simulink model "synchro_v3"  (R2020b)
settings: Solver=FixedStepAuto  StartTime=0.0  StopTime=2  FixedStep=Ts  RelTol=1e-3
values from neighbouring files (symbols this model uses):
  m = 5/100    (= 0.05)    [synchro_parameters_v1.m]
  Sbase = 1    [synchro_parameters_v1.m]
  Ts = 1/Fs    (= 0.0001)    [synchro_parameters_v1.m]
  Vbase = 1    [synchro_parameters_v1.m]
  w_droop = 10*2*pi    (= 62.8318530718)    [synchro_parameters_v1.m]
  w_pll = 10*2*pi    (= 62.8318530718)    [synchro_parameters_v1.m]
  w_tau = 1e3*2*pi    (= 6283.18530718)    [synchro_parameters_v1.m]
  Wbase = 2*pi*50    (= 314.159265359)    [synchro_parameters_v1.m]
  Ybase = 1/Zbase    (= 1)    [synchro_parameters_v1.m]
  Zbase = Vbase/Ibase    (= 1)    [synchro_parameters_v1.m]
undefined symbols (not defined in the file or in its folder): DiscIntNeverNeededParam
libraries: SimplexPS x69, powerlib x64
(part 1 of 2)
settings Model: Creator=admin_user  LastModifiedBy=admin_user

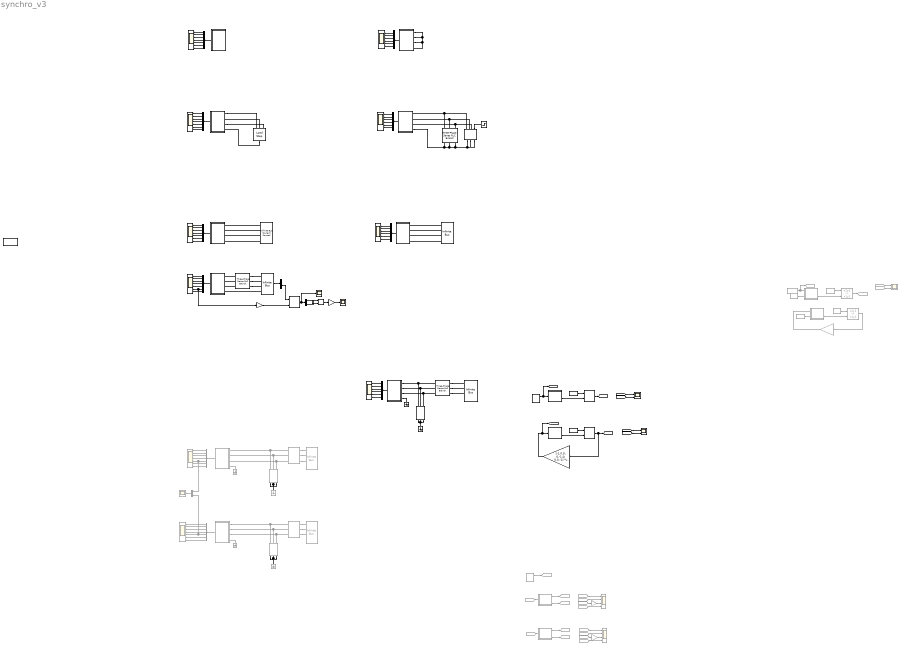
== system synchro_v3 ==
  note: Single-Inverter-Load System
  note: Droop inverter & voltage-source infinite bus
  note: PLL inverter & voltage-source infinite bus
  note: Droop inverter & current-source infinite bus
  note: Single-Inverter-Infinite-Bus System
  note: dq frame analysis
  note: PLL inverter + inifinite voltage bus (dq frame)
  note: PLL inverter + infinite voltage bus
  note: Droop analysis
  note: PLL analysis
  note: i-type
  note: Droop Inverter
  note: PLL inverter + R load
  note: PLL inverter & current-source infinite bus
  note: Droop inverter & R load
  note: PLL inverter & R load
  note: PLL inverter & R load
  note: Single-Inverter Extreme Operation
  note: Droop inverter & R load
  Atan : Trigonometry  Operator=atan2
  Bus Selector{,5,7,9} (4 alike) : BusSelector  OutputSignals=v_dq,i_dq,v_abc,i_abc,w,theta,pq
  Bus Selector1 : BusSelector  Commented=on  OutputSignals=v_dq,i_dq,v_abc,i_abc,w,theta,pq
  Bus Selector{3..4,8,10} (4 alike) : BusSelector  OutputSignals=v_dq,i_dq,v_abc,i_abc,w,theta
  Bus Selector2 : BusSelector  Commented=on  OutputSignals=v_dq,i_dq,v_abc,i_abc,w,theta,pq
  Bus Selector6 : BusSelector  OutputSignals=v_dq,v_abc
  Constant : Constant  Value=[1 0]
  Constant1 : Constant  Commented=on  Value=[1 0]
  Constant2 : Constant  Commented=on  Value=Wbase
  Constant3 : Constant  Commented=on  Value=[1 0]
  Constant4 : Constant  Value=[0.5 -0.1]
  Constant5 : Constant  Commented=on  Value=Wbase
  Constant6 : Constant  Commented=on  Value=[1;0]
  Demux : Demux  Outputs=2
  Droop Inverter : Subsystem
  Droop Inverter1 : Subsystem
  Droop Inverter2 : Subsystem
  Droop Inverter3 : Subsystem
  Frequency Droop (id) : Subsystem  Commented=on  AncestorBlock=SimplexPS/Frequency Droop (id)  mask{Ts=Ts, Sbase=Sbase, Vbase=Vbase, Wbase=Wbase, m=m, w_tau=w_droop, theta0=0, P0=0, W0=1}
      mask prompts: Ts "Ts (s), samping period"; Sbase "Sbase (VA), base power"; Vbase "Vbase (V), base voltage"; Wbase "Wbase (rad/s), base angular frequency"; m "m (pu), droop gain"; w_tau "w_tau (rad/s), low-pass filter bandwidth"; theta0 "theta0 (rad), initial angle"; P0 "P0 (pu), power setting point"; W0 "W0 (pu), frequency setting point"
  Frequency Droop (iq) : Subsystem  Commented=on  AncestorBlock=SimplexPS/Frequency Droop (iq)  mask{Ts=Ts, Sbase=Sbase, Vbase=Vbase, Wbase=Wbase, m=m, w_tau=w_droop, theta0=0, P0=0, W0=1}
      mask prompts: Ts "Ts (s), samping period"; Sbase "Sbase (VA), base power"; Vbase "Vbase (V), base voltage"; Wbase "Wbase (rad/s), base angular frequency"; m "m (pu), droop gain"; w_tau "w_tau (rad/s), low-pass filter bandwidth"; theta0 "theta0 (rad), initial angle"; P0 "P0 (pu), power setting point"; W0 "W0 (pu), frequency setting point"
  From{9..10,12,14} (4 alike) : From  Commented=on  GotoTag=i_abc3
  From11 : From  Commented=on  GotoTag=v_abc3
  From15 : From  Commented=on  GotoTag=v_abc4
  From16 : From  Commented=on  GotoTag=w4
  From17 : From  Commented=on  GotoTag=theta4
  From2 : From  Commented=on  GotoTag=vDQ_PLL
  From3 : From  Commented=on  GotoTag=iDQ_PLL
  From6 : From  Commented=on  GotoTag=w3
  From7 : From  Commented=on  GotoTag=theta3
  Gain : Gain  Commented=on  Gain=[0.5,0;0,0.5]  Multiplication=Matrix(K*u)
  Gain1 : Gain  Commented=on  Gain=1/Wbase
  Gain2 : Gain  Commented=on  Gain=1/Wbase
  Gain3 : Gain  Gain=[-1,0,0; 0,-1,0; 0,0,-1]  Multiplication=Matrix(K*u)
  Gain4 : Gain  Gain=2*pi
  Gain5 : Gain  Gain=1/(2*pi)
  Goto10 : Goto  Commented=on  GotoTag=theta4
  Goto2 : Goto  Commented=on  GotoTag=iDQ_PLL
  Goto3 : Goto  Commented=on  GotoTag=vDQ_PLL
  Goto5 : Goto  Commented=on  GotoTag=w3
  Goto6 : Goto  Commented=on  GotoTag=theta3
  Goto7 : Goto  Commented=on  GotoTag=i_abc3
  Goto9 : Goto  Commented=on  GotoTag=w4
  Ground{2..5} (4 alike) : powerlib/Elements/Ground  Commented=on  LConnTagsString=a
  Ground6 : powerlib/Elements/Ground  LConnTagsString=a
  Ground8 : powerlib/Elements/Ground  LConnTagsString=a
  Infinite Bus : SimplexPS/Infinite Bus  Commented=on  Ts=Ts  Sbase=Sbase  Vbase=Vbase  Wbase=Wbase  vd=1  vq=0  theta0=0  w=Wbase  R=1e-30
      settings: SourceProductName=Simplex Power Systems
  Infinite Bus (Current Source) : SimplexPS/Infinite Bus (Current Source)  Ts=Ts  Sbase=Sbase  Vbase=Vbase  Wbase=Wbase  id=1  iq=0  theta0=0  w=0.98
      settings: SourceProductName=Simplex Power Systems
  Infinite Bus1 : SimplexPS/Infinite Bus  Commented=on  Ts=Ts  Sbase=Sbase  Vbase=Vbase  Wbase=Wbase  vd=1  vq=0  theta0=0  w=Wbase  R=1e-30
      settings: SourceProductName=Simplex Power Systems
  Infinite Bus2 : SimplexPS/Infinite Bus  Ts=Ts  Sbase=Sbase  Vbase=Vbase  Wbase=Wbase  vd=1  vq=0  theta0=0  w=Wbase  R=1e-30
      settings: SourceProductName=Simplex Power Systems
  Infinite Bus3 : SimplexPS/Infinite Bus  Ts=Ts  Sbase=Sbase  Vbase=Vbase  Wbase=Wbase  vd=1  vq=0  theta0=0  w=Wbase  R=1e-30
      settings: SourceProductName=Simplex Power Systems
  Infinite Bus4 : SimplexPS/Infinite Bus  Ts=Ts  Sbase=Sbase  Vbase=Vbase  Wbase=Wbase  vd=1.01  vq=0  theta0=0  w=Wbase  R=1e-30
      settings: SourceProductName=Simplex Power Systems
  Load Step1 : SimplexPS/Load Step  t0=1  R=2*Zbase  Reverse=0
      settings: SourceProductName=Simplex Power Systems
  Mux : Mux  Commented=on  Inputs=2
  "PLL (vDQ -> vq)" : Subsystem  Commented=on  AncestorBlock=|  mask{Ts=Ts, Vbase=Vbase, Wbase=Wbase, w_PLL=w_pll, w_tau=w_tau, theta0=0}
      | SimplexPS/PLL
      | (vDQ -> vq)
      mask prompts: Ts "Ts (s), sampling period"; Vbase "Vbase (V), base voltage"; Wbase "Wbase (rad/s), base angular frequency"; w_PLL "w_pll (rad/s), PLL bandwidth"; w_tau "w_tau (rad/s), low-pass filter bandwidth"; theta0 "theta0 (rad), initial angle"
  "PLL (vDQ -> vq)1" : Subsystem  Commented=on  AncestorBlock=|  mask{Ts=Ts, Vbase=Vbase, Wbase=Wbase, w_PLL=w_pll, w_tau=w_tau, theta0=pi/2}
      | SimplexPS/PLL
      | (vDQ -> vq)
      mask prompts: Ts "Ts (s), sampling period"; Vbase "Vbase (V), base voltage"; Wbase "Wbase (rad/s), base angular frequency"; w_PLL "w_pll (rad/s), PLL bandwidth"; w_tau "w_tau (rad/s), low-pass filter bandwidth"; theta0 "theta0 (rad), initial angle"
  "PLL (vabc -> vq)" : Subsystem  AncestorBlock=|  mask{Ts=Ts, Vbase=Vbase, Wbase=Wbase, w_pll=w_pll, w_tau=w_tau, theta0=0}
      | SimplexPS/PLL
      | (vabc -> vq)
      mask prompts: Ts "Ts (s), sampling period"; Vbase "Vbase (V), base voltage"; Wbase "Wbase (rad/s), base angular frequency"; w_pll "w_pll (rad/s), PLL bandwidth"; w_tau "w_tau (rad/s), low-pass filter bandwidth"; theta0 "theta0 (rad), initial angle"
  "PLL (vabc -> vq)1" : Subsystem  AncestorBlock=|  mask{Ts=Ts, Vbase=Vbase, Wbase=Wbase, w_pll=w_pll, w_tau=w_tau, theta0=pi/2/2}
      | SimplexPS/PLL
      | (vabc -> vq)
      mask prompts: Ts "Ts (s), sampling period"; Vbase "Vbase (V), base voltage"; Wbase "Wbase (rad/s), base angular frequency"; w_pll "w_pll (rad/s), PLL bandwidth"; w_tau "w_tau (rad/s), low-pass filter bandwidth"; theta0 "theta0 (rad), initial angle"
  PLL Inverter : Subsystem
  PLL Inverter1 : Subsystem
  PLL Inverter2 : Subsystem
  PLL Inverter3 : Subsystem
  Scope{,11,14,16} (4 alike) : Scope  NumInputPorts=7
  Scope1 : Scope  NumInputPorts=2
  Scope{4,10,15,17} (4 alike) : Scope  NumInputPorts=6
  Scope12 : Scope
  Scope13 : Scope
  Scope2 : Scope  Commented=on  NumInputPorts=4
  Scope3 : Scope  Commented=on  NumInputPorts=7
  Scope5 : Scope  Commented=on  NumInputPorts=7
  Scope6 : Scope  Commented=on
  Scope7 : Scope  Commented=on  NumInputPorts=4
  Scope8 : Scope  Commented=on  NumInputPorts=2
  Scope9 : Scope  NumInputPorts=2
  Step : Step  SampleTime=0
  Three-Phase Parallel RLC Branch1 : powerlib/Elements/Three-Phase Parallel RLC Branch  Commented=on  LConnTagsString=A|B|C  RConnTagsString=A|B|C  BranchType=R  Resistance=1  Inductance=1e-3  Capacitance=1e-6  Measurements=None
      settings: SourceProductBaseCode=PS
  Three-Phase Parallel RLC Branch2 : powerlib/Elements/Three-Phase Parallel RLC Branch  Commented=on  LConnTagsString=A|B|C  RConnTagsString=A|B|C  BranchType=R  Resistance=1  Inductance=1e-3  Capacitance=1e-6  Measurements=None
      settings: SourceProductBaseCode=PS
  Three-Phase Series RLC Branch1 : powerlib/Elements/Three-Phase Series RLC Branch  LConnTagsString=A|B|C  RConnTagsString=A|B|C  BranchType=C  Resistance=1  Inductance=0.2/(2*pi*50)  Capacitance=Ybase*1e-3/Wbase  Measurements=None
  Three-Phase Series RLC Branch2 : powerlib/Elements/Three-Phase Series RLC Branch  Commented=on  LConnTagsString=A|B|C  RConnTagsString=A|B|C  BranchType=RL  Resistance=0.01  Inductance=0.2/(2*pi*50)  Capacitance=1e-6  Measurements=None
  Three-Phase Series RLC Branch3 : powerlib/Elements/Three-Phase Series RLC Branch  Commented=on  LConnTagsString=A|B|C  RConnTagsString=A|B|C  BranchType=RL  Resistance=0.01  Inductance=0.2/(2*pi*50)  Capacitance=1e-6  Measurements=None
  Three-Phase Series RLC Branch4 : powerlib/Elements/Three-Phase Series RLC Branch  LConnTagsString=A|B|C  RConnTagsString=A|B|C  BranchType=RL  Resistance=0.01*Zbase*0.4  Inductance=0.3*Zbase/Wbase*0.4  Capacitance=1/Wbase  Measurements=None
  Three-Phase Series RLC Branch5 : powerlib/Elements/Three-Phase Series RLC Branch  LConnTagsString=A|B|C  RConnTagsString=A|B|C  BranchType=RL  Resistance=0.3*Zbase/5  Inductance=0.3*Zbase/Wbase  Capacitance=1/Wbase  Measurements=None
  Three-Phase Series RLC Branch7 : powerlib/Elements/Three-Phase Series RLC Branch  LConnTagsString=A|B|C  RConnTagsString=A|B|C  BranchType=R  Resistance=2*Zbase  Inductance=0.3*Zbase/Wbase  Capacitance=1/Wbase  Measurements=None
  Three-Phase Breaker : powerlib/Elements/Three-Phase Breaker  InitialState=open  SwitchA=on  SwitchB=on  SwitchC=on  SwitchTimes="[1/60  5/60]"  External=on  BreakerResistance=1e-9  SnubberResistance=1e6  SnubberCapacitance=inf  Measurements=None
  Three-Phase Signal : SimplexPS/Three-Phase Signal  Commented=on  ud=1  uq=0  w=Wbase*1  theta0=0
      settings: SourceProductName=Simplex Power Systems
  Three-Phase Signal1 : SimplexPS/Three-Phase Signal  ud=1  uq=0  w=Wbase*0.95  theta0=pi/2/2
      settings: SourceProductName=Simplex Power Systems
  Voltage-Type Inverter (Droop)1 : Subsystem  Commented=on  mask{Sbase=Sbase, Vbase=Vbase, Wbase=Wbase, Ts=Ts, v_d0=1, v_q0=0, w0=1, m=m, n=0, P0=0, Q0=0, w_droop=w_droop}
      mask prompts: Sbase "Sbase (VA)"; Vbase "Vbase (V)"; Wbase "Wbase (rad/s)"; Ts "Ts (s)"; v_d0 "v_d0 (pu), d-axis voltage setting point"; v_q0 "v_q0 (pu), q-axis voltage setting point"; w0 "w0 (pu), frequency setting point"; m "m (pu), frequency droop gain"; n "n (pu), voltage droop gain"; P0 "P0 (pu), active power setting point"; Q0 "Q0 (pu), reactive power setting point"; w_droop "w_droop (rad/s), droop bandwidth"
  Voltage-Type Inverter (Droop)2 : Subsystem  Commented=on  mask{Sbase=Sbase, Vbase=Vbase, Wbase=Wbase, Ts=Ts, v_d0=1, v_q0=0, w0=1, m=m, n=0, P0=0, Q0=0, w_droop=w_droop}
      mask prompts: Sbase "Sbase (VA)"; Vbase "Vbase (V)"; Wbase "Wbase (rad/s)"; Ts "Ts (s)"; v_d0 "v_d0 (pu), d-axis voltage setting point"; v_q0 "v_q0 (pu), q-axis voltage setting point"; w0 "w0 (pu), frequency setting point"; m "m (pu), frequency droop gain"; n "n (pu), voltage droop gain"; P0 "P0 (pu), active power setting point"; Q0 "Q0 (pu), reactive power setting point"; w_droop "w_droop (rad/s), droop bandwidth"
  "abc -> dq (Power-Invariant)" : SimplexPS/abc -> dq (Power-Invariant)  SystemSampleTime=-1  VariantActivationTime=update diagram  Latency=0  AutoFrameSizeCalculation=off
      settings: SourceProductName=Simplex Power Systems
  "dq -> abc (Power-Invariant)" : SimplexPS/dq -> abc (Power-Invariant)  SystemSampleTime=-1  VariantActivationTime=update diagram  Latency=0  AutoFrameSizeCalculation=off
      settings: SourceProductName=Simplex Power Systems
  "dq -> abc (Power-Invariant)1" : SimplexPS/dq -> abc (Power-Invariant)  SystemSampleTime=-1  VariantActivationTime=update diagram  Latency=0  AutoFrameSizeCalculation=off
      settings: SourceProductName=Simplex Power Systems
  powergui : powerlib/powergui  Priority=1  SimulationMode=Discrete  SampleTime=Ts  frequency=60  Iterations=50  frequencyindice=0  Pbase=100e6  ErrMax=1e-4  UnitsV=kV  UnitsW=MW  buscounter=0  FunctionMessages=off  echomessages=off  EnableUseOfTLC=off  CurrentSourceSwitches=off  DisableSnubberDevices=off  DisableRonSwitches=off  DisableVfSwitches=off  DisplayEquations=off  AutomaticDiscreteSolvers=off  SolverType=Tustin/Backward Euler (TBE)  Interpol=off  ExternalGateDelay=off  methode=off  Ts=100  x0status=blocks  SPID=on  SwTol=0  HookPort=off  NonlinearTolerance=1e-4  nMaxIteration=100  ContinueOnMaxIteration=off  RestoreLinks=warning  ResistiveCurrentMeasurement=off  Frange=[0:2:500]  Ylog=off  Xlog=on  ShowGrid=off  save=off  variable=ZData  structure=0  ZoomFFT=off  StartTime=0.0  cycles=1  DisplayStyle=1  fundamental=60  FreqAxis=off  MaxFrequency=1000  frequencyindicesteady=1  RmsSteady=1  display=off
  "x2y2 -> x1y1" : SimplexPS/x2y2 -> x1y1  Commented=on  SystemSampleTime=-1  VariantActivationTime=update diagram  Latency=0  AutoFrameSizeCalculation=off
      settings: SourceProductName=Simplex Power Systems
  "x2y2 -> x1y2" : SimplexPS/x2y2 -> x1y1  Commented=on  SystemSampleTime=-1  VariantActivationTime=update diagram  Latency=0  AutoFrameSizeCalculation=off
      settings: SourceProductName=Simplex Power Systems
  wires:
  Droop Inverter/1(m) -> Bus Selector/1
  Bus Selector/1 -> Scope/1  "<v_dq>"
  Bus Selector/2 -> Scope/2  "<i_dq>"
  Bus Selector/3 -> Scope/3  "<v_abc>"
  Bus Selector/4 -> Scope/4  "<i_abc>"
  Bus Selector/5 -> Scope/5  "<w>"
  Bus Selector/6 -> Scope/6  "<theta>"
  Bus Selector/7 -> Scope/7  "<pq>"
  Bus Selector4/3 -> Scope4/3  "<v_abc>"
  Bus Selector4/4 -> Scope4/4  "<i_abc>"
  Bus Selector4/6 -> Scope4/6  "<theta>"
  Bus Selector4/1 -> Scope4/1  "<v_dq>"
  PLL Inverter/1(m) -> Bus Selector4/1
  Bus Selector4/5 -> Scope4/5  "<w>"
  Bus Selector4/2 -> Scope4/2  "<i_dq>"
  Frequency Droop (id)/1(w) -> Goto5/1
  Frequency Droop (id)/3(theta) -> Goto6/1
  From7/1 -> Scope2/4
  Three-Phase Signal/1 -> Goto7/1
  From9/1 -> Frequency Droop (id)/1(iabc)
  From10/1 -> Scope2/1
  From11/1 -> Scope2/2
  From6/1 -> Gain1/1
  Gain1/1 -> Scope2/3
  Bus Selector1/5 -> Mux/1, Scope3/5  "<w>"
  Bus Selector1/3 -> Scope3/3  "<v_abc>"
  Bus Selector1/6 -> Scope3/6  "<theta>"
  Bus Selector1/7 -> Scope3/7  "<pq>"
  Bus Selector1/2 -> Scope3/2  "<i_dq>"
  Bus Selector1/4 -> Scope3/4  "<i_abc>"
  Bus Selector1/1 -> Scope3/1  "<v_dq>"
  Voltage-Type Inverter (Droop)1/1(m) -> Bus Selector1/1
  Bus Selector2/2 -> Scope5/2  "<i_dq>"
  Bus Selector2/4 -> Scope5/4  "<i_abc>"
  Bus Selector2/1 -> Scope5/1  "<v_dq>"
  Voltage-Type Inverter (Droop)2/1(m) -> Bus Selector2/1
  Bus Selector2/6 -> Scope5/6  "<theta>"
  Bus Selector2/3 -> Scope5/3  "<v_abc>"
  Bus Selector2/7 -> Scope5/7  "<pq>"
  Bus Selector2/5 -> Mux/2, Scope5/5  "<w>"
  Mux/1 -> Scope6/1
  From12/1 -> Frequency Droop (iq)/1(iabc)
  Frequency Droop (iq)/1(w) -> Goto9/1
  Frequency Droop (iq)/3(theta) -> Goto10/1
  From17/1 -> Scope7/4
  From16/1 -> Gain2/1
  From15/1 -> Scope7/2
  From14/1 -> Scope7/1
  Gain2/1 -> Scope7/3
  Three-Phase Signal1/1 -> "PLL (vabc -> vq)"/1(vabc), [vabc_PLL1]
  Constant/1 -> "dq -> abc (Power-Invariant)"/1
  "PLL (vabc -> vq)"/2(theta) -> "dq -> abc (Power-Invariant)"/2
  "dq -> abc (Power-Invariant)"/1 -> [iabc_PLL1]
  [iabc_PLL1] -> Scope1/2
  [vabc_PLL1] -> Scope1/1
  Constant2/1 -> "PLL (vDQ -> vq)"/2(wDQ)
  Constant3/1 -> "x2y2 -> x1y1"/1
  "PLL (vDQ -> vq)"/2(theta) -> "x2y2 -> x1y1"/2
  "x2y2 -> x1y1"/1 -> Goto2/1
  Constant1/1 -> "PLL (vDQ -> vq)"/1(vDQ), Goto3/1
  From2/1 -> Scope8/1
  From3/1 -> Scope8/2
  Constant6/1 -> "x2y2 -> x1y2"/1
  "PLL (vDQ -> vq)1"/2(theta) -> "x2y2 -> x1y2"/2
  "x2y2 -> x1y2"/1 -> Gain/1
  Constant5/1 -> "PLL (vDQ -> vq)1"/2(wDQ)
  Gain/1 -> "PLL (vDQ -> vq)1"/1(vDQ)
  "PLL (vabc -> vq)1"/2(theta) -> "dq -> abc (Power-Invariant)1"/2
  [vabc_PLL2] -> Scope9/1
  Constant4/1 -> "dq -> abc (Power-Invariant)1"/1
  Gain3/1 -> [vabc_PLL2], "PLL (vabc -> vq)1"/1(vabc)
  [iabc_PLL2] -> Scope9/2
  "dq -> abc (Power-Invariant)1"/1 -> [iabc_PLL2], Gain3/1
  Bus Selector3/3 -> Scope10/3  "<v_abc>"
  Bus Selector3/1 -> Scope10/1  "<v_dq>"
  Bus Selector3/6 -> Scope10/6  "<theta>"
  Bus Selector3/5 -> Scope10/5  "<w>"
  Bus Selector3/4 -> Scope10/4  "<i_abc>"
  PLL Inverter1/1(m) -> Bus Selector3/1
  Bus Selector3/2 -> Scope10/2  "<i_dq>"
  Bus Selector5/1 -> Scope11/1  "<v_dq>"
  Bus Selector5/6 -> Gain4/1, Scope11/6  "<theta>"
  Bus Selector5/2 -> Scope11/2  "<i_dq>"
  Bus Selector5/4 -> Scope11/4  "<i_abc>"
  Droop Inverter1/1(m) -> Bus Selector5/1
  Bus Selector5/7 -> Scope11/7  "<pq>"
  Bus Selector5/5 -> Scope11/5  "<w>"
  Bus Selector5/3 -> Scope11/3  "<v_abc>"
  Infinite Bus4/1 -> Bus Selector6/1
  Bus Selector6/2 -> "abc -> dq (Power-Invariant)"/1  "<v_abc>"
  Demux/1 -> Atan/2
  Demux/2 -> Atan/1
  "abc -> dq (Power-Invariant)"/1 -> Scope13/1, Demux/1
  Gain4/1 -> "abc -> dq (Power-Invariant)"/2
  Atan/1 -> Gain5/1
  Gain5/1 -> Scope12/1
  Bus Selector7/3 -> Scope14/3  "<v_abc>"
  Bus Selector7/6 -> Scope14/6  "<theta>"
  Bus Selector7/2 -> Scope14/2  "<i_dq>"
  Bus Selector7/1 -> Scope14/1  "<v_dq>"
  Droop Inverter2/1(m) -> Bus Selector7/1
  Bus Selector7/7 -> Scope14/7  "<pq>"
  Bus Selector7/5 -> Scope14/5  "<w>"
  Bus Selector7/4 -> Scope14/4  "<i_abc>"
  PLL Inverter2/1(m) -> Bus Selector8/1
  Bus Selector8/2 -> Scope15/2  "<i_dq>"
  Bus Selector8/1 -> Scope15/1  "<v_dq>"
  Bus Selector8/4 -> Scope15/4  "<i_abc>"
  Bus Selector8/3 -> Scope15/3  "<v_abc>"
  Bus Selector8/6 -> Scope15/6  "<theta>"
  Bus Selector8/5 -> Scope15/5  "<w>"
  Bus Selector10/4 -> Scope17/4  "<i_abc>"
  Bus Selector10/5 -> Scope17/5  "<w>"
  PLL Inverter3/1(m) -> Bus Selector10/1
  Bus Selector9/5 -> Scope16/5  "<w>"
  Bus Selector9/1 -> Scope16/1  "<v_dq>"
  Bus Selector10/6 -> Scope17/6  "<theta>"
  Bus Selector9/7 -> Scope16/7  "<pq>"
  Bus Selector9/2 -> Scope16/2  "<i_dq>"
  Bus Selector10/1 -> Scope17/1  "<v_dq>"
  Bus Selector9/4 -> Scope16/4  "<i_abc>"
  Droop Inverter3/1(m) -> Bus Selector9/1
  Bus Selector9/6 -> Scope16/6  "<theta>"
  Bus Selector9/3 -> Scope16/3  "<v_abc>"
  Bus Selector10/2 -> Scope17/2  "<i_dq>"
  Bus Selector10/3 -> Scope17/3  "<v_abc>"
  Step/1 -> Three-Phase Breaker/1
  connections:
  Infinite Bus (Current Source)/LConn1 -- Droop Inverter/LConn1
  Infinite Bus (Current Source)/LConn2 -- Droop Inverter/LConn2
  Infinite Bus (Current Source)/LConn3 -- Droop Inverter/LConn3
  PLL Inverter/LConn4 -- Ground8/LConn1
  Three-Phase Parallel RLC Branch1/RConn2 -- Ground2/LConn1 -- Three-Phase Parallel RLC Branch1/RConn3 -- Three-Phase Parallel RLC Branch1/RConn1
  Three-Phase Parallel RLC Branch1/LConn3 -- Voltage-Type Inverter (Droop)1/LConn3 -- Three-Phase Series RLC Branch3/LConn3
  Ground3/LConn1 -- Voltage-Type Inverter (Droop)1/LConn4
  Three-Phase Parallel RLC Branch1/LConn2 -- Voltage-Type Inverter (Droop)1/LConn2 -- Three-Phase Series RLC Branch3/LConn2
  Three-Phase Parallel RLC Branch1/LConn1 -- Voltage-Type Inverter (Droop)1/LConn1 -- Three-Phase Series RLC Branch3/LConn1
  Three-Phase Parallel RLC Branch2/RConn2 -- Ground4/LConn1 -- Three-Phase Parallel RLC Branch2/RConn3 -- Three-Phase Parallel RLC Branch2/RConn1
  Voltage-Type Inverter (Droop)2/LConn3 -- Three-Phase Series RLC Branch2/LConn3 -- Three-Phase Parallel RLC Branch2/LConn3
  Ground5/LConn1 -- Voltage-Type Inverter (Droop)2/LConn4
  Voltage-Type Inverter (Droop)2/LConn1 -- Three-Phase Parallel RLC Branch2/LConn1 -- Three-Phase Series RLC Branch2/LConn1
  Voltage-Type Inverter (Droop)2/LConn2 -- Three-Phase Series RLC Branch2/LConn2 -- Three-Phase Parallel RLC Branch2/LConn2
  Three-Phase Series RLC Branch2/RConn1 -- Infinite Bus/LConn1
  Three-Phase Series RLC Branch2/RConn2 -- Infinite Bus/LConn2
  Three-Phase Series RLC Branch2/RConn3 -- Infinite Bus/LConn3
  Three-Phase Series RLC Branch3/RConn1 -- Infinite Bus1/LConn1
  Three-Phase Series RLC Branch3/RConn3 -- Infinite Bus1/LConn3
  Three-Phase Series RLC Branch3/RConn2 -- Infinite Bus1/LConn2
  Ground6/LConn1 -- Three-Phase Series RLC Branch1/RConn3 -- Three-Phase Series RLC Branch1/RConn2 -- Three-Phase Series RLC Branch1/RConn1
  PLL Inverter/LConn1 -- Three-Phase Series RLC Branch1/LConn1 -- Three-Phase Series RLC Branch4/RConn1
  PLL Inverter/LConn2 -- Three-Phase Series RLC Branch1/LConn2 -- Three-Phase Series RLC Branch4/RConn2
  PLL Inverter/LConn3 -- Three-Phase Series RLC Branch4/RConn3 -- Three-Phase Series RLC Branch1/LConn3
  Three-Phase Series RLC Branch4/LConn1 -- Infinite Bus2/LConn1
  Three-Phase Series RLC Branch4/LConn2 -- Infinite Bus2/LConn2
  Three-Phase Series RLC Branch4/LConn3 -- Infinite Bus2/LConn3
  Infinite Bus3/LConn1 -- PLL Inverter1/LConn1
  Infinite Bus3/LConn2 -- PLL Inverter1/LConn2
  Infinite Bus3/LConn3 -- PLL Inverter1/LConn3
  Infinite Bus3/LConn4 -- PLL Inverter1/LConn4
  Infinite Bus (Current Source)/LConn4 -- Droop Inverter/LConn4
  Infinite Bus4/LConn4 -- Droop Inverter1/LConn4
  Three-Phase Series RLC Branch5/RConn1 -- Droop Inverter1/LConn1
  Three-Phase Series RLC Branch5/RConn2 -- Droop Inverter1/LConn2
  Three-Phase Series RLC Branch5/RConn3 -- Droop Inverter1/LConn3
  Three-Phase Series RLC Branch5/LConn1 -- Infinite Bus4/LConn1
  Three-Phase Series RLC Branch5/LConn2 -- Infinite Bus4/LConn2
  Three-Phase Series RLC Branch5/LConn3 -- Infinite Bus4/LConn3
  Droop Inverter2/LConn1 -- Load Step1/LConn1
  Load Step1/LConn2 -- Droop Inverter2/LConn2
  Droop Inverter2/LConn3 -- Load Step1/LConn3
  Load Step1/RConn1 -- Droop Inverter2/LConn4
  Three-Phase Series RLC Branch7/RConn1 -- Three-Phase Breaker/LConn3 -- PLL Inverter2/LConn1
  Three-Phase Series RLC Branch7/RConn2 -- Three-Phase Breaker/LConn2 -- PLL Inverter2/LConn2
  Three-Phase Series RLC Branch7/RConn3 -- Three-Phase Breaker/LConn1 -- PLL Inverter2/LConn3
  PLL Inverter2/LConn4 -- Three-Phase Breaker/RConn1 -- Three-Phase Breaker/RConn2 -- Three-Phase Breaker/RConn3 -- Three-Phase Series RLC Branch7/LConn3 -- Three-Phase Series RLC Branch7/LConn2 -- Three-Phase Series RLC Branch7/LConn1
  PLL Inverter3/LConn1 -- PLL Inverter3/LConn2 -- PLL Inverter3/LConn3 -- PLL Inverter3/LConn4

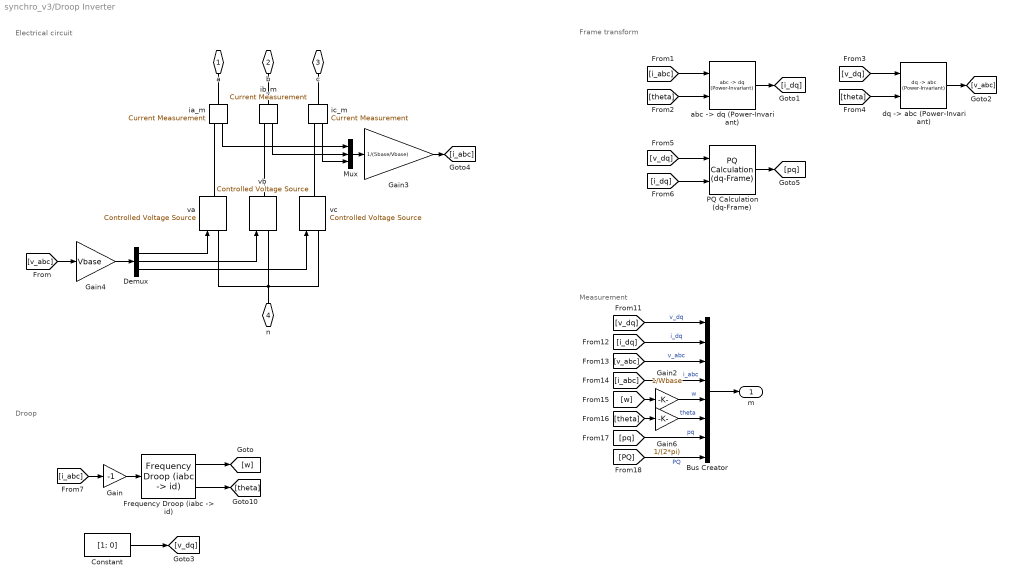
== system synchro_v3/Droop Inverter ==
  note: Measurement
  note: Droop
  note: Frame transform
  note: Electrical circuit
  Bus Creator : BusCreator  Inputs=8
  Constant : Constant  Value=[1; 0]
  Demux : Demux  Outputs=3
  "Frequency Droop (iabc -> id)" : SimplexPS/Frequency Droop (iabc -> id)  Ts=Ts  Sbase=Sbase  Vbase=Vbase  Wbase=Wbase  m=m  w_tau=w_droop  theta0=0  i0=0  w0=1
      settings: SourceProductName=Simplex Power Systems
  Gain : Gain  Gain=-1
  Gain2 : Gain  Gain=1/Wbase
  Gain3 : Gain  Gain=1/(Sbase/Vbase)
  Gain4 : Gain  Gain=Vbase
  Gain6 : Gain  Gain=1/(2*pi)
  Mux : Mux  Inputs=3
  PQ Calculation (dq-Frame) : SimplexPS/PQ Calculation (dq-Frame)  SystemSampleTime=-1  VariantActivationTime=update diagram  Latency=0  AutoFrameSizeCalculation=off
      settings: SourceProductName=Simplex Power Systems
  "abc -> dq (Power-Invariant)" : SimplexPS/abc -> dq (Power-Invariant)  SystemSampleTime=-1  VariantActivationTime=update diagram  Latency=0  AutoFrameSizeCalculation=off
      settings: SourceProductName=Simplex Power Systems
  "dq -> abc (Power-Invariant)" : SimplexPS/dq -> abc (Power-Invariant)  SystemSampleTime=-1  VariantActivationTime=update diagram  Latency=0  AutoFrameSizeCalculation=off
      settings: SourceProductName=Simplex Power Systems
  ia_m : powerlib/Measurements/Current Measurement  PhasorSimulation=off  OutputType=Complex  PSBequivalent=0
  ib_m : powerlib/Measurements/Current Measurement  PhasorSimulation=off  OutputType=Complex  PSBequivalent=0
  ic_m : powerlib/Measurements/Current Measurement  PhasorSimulation=off  OutputType=Complex  PSBequivalent=0
  va : powerlib/Electrical Sources/Controlled Voltage Source  Initialize=on  Source_Type=AC  Amplitude=0  Phase=0  Frequency=0  Measurements=None
  vb : powerlib/Electrical Sources/Controlled Voltage Source  Initialize=on  Source_Type=AC  Amplitude=0  Phase=0  Frequency=0  Measurements=None
  vc : powerlib/Electrical Sources/Controlled Voltage Source  Initialize=on  Source_Type=AC  Amplitude=0  Phase=0  Frequency=0  Measurements=None
  a : PMIOPort  Side=Left
  b : PMIOPort  Port=2  Side=Left
  c : PMIOPort  Port=3  Side=Left
  n : PMIOPort  Port=4  Side=Left
  m : Outport
  wires:
  ic_m/1 -> Mux/3
  ia_m/1 -> Mux/1
  ib_m/1 -> Mux/2
  Demux/1 -> va/1
  Demux/2 -> vb/1
  Demux/3 -> vc/1
  [i_abc] -> "abc -> dq (Power-Invariant)"/1
  [theta] -> "abc -> dq (Power-Invariant)"/2
  "abc -> dq (Power-Invariant)"/1 -> [i_dq]
  [v_dq] -> "dq -> abc (Power-Invariant)"/1
  [theta] -> "dq -> abc (Power-Invariant)"/2
  "dq -> abc (Power-Invariant)"/1 -> [v_abc]
  [v_dq] -> Bus Creator/1  "v_dq"
  [v_abc] -> Bus Creator/3  "v_abc"
  [i_abc] -> Bus Creator/4  "i_abc"
  [pq] -> Bus Creator/7  "pq"
  [PQ] -> Bus Creator/8  "PQ"
  Bus Creator/1 -> m/1
  [w] -> Gain2/1
  Gain2/1 -> Bus Creator/5  "w"
  Mux/1 -> Gain3/1
  Gain3/1 -> [i_abc]
  [v_abc] -> Gain4/1
  Gain4/1 -> Demux/1
  [theta] -> Gain6/1
  Gain6/1 -> Bus Creator/6  "theta"
  "Frequency Droop (iabc -> id)"/2 -> [theta]
  [i_abc] -> Gain/1
  "Frequency Droop (iabc -> id)"/1 -> [w]
  Constant/1 -> [v_dq]
  [i_dq] -> Bus Creator/2  "i_dq"
  [v_dq] -> PQ Calculation (dq-Frame)/1
  [i_dq] -> PQ Calculation (dq-Frame)/2
  PQ Calculation (dq-Frame)/1 -> [pq]
  Gain/1 -> "Frequency Droop (iabc -> id)"/1
  connections:
  ia_m/RConn1 -- va/RConn1
  ia_m/LConn1 -- a/RConn1
  ib_m/RConn1 -- vb/RConn1
  ic_m/RConn1 -- vc/RConn1
  va/LConn1 -- vb/LConn1 -- vc/LConn1 -- n/RConn1
  ib_m/LConn1 -- b/RConn1
  ic_m/LConn1 -- c/RConn1

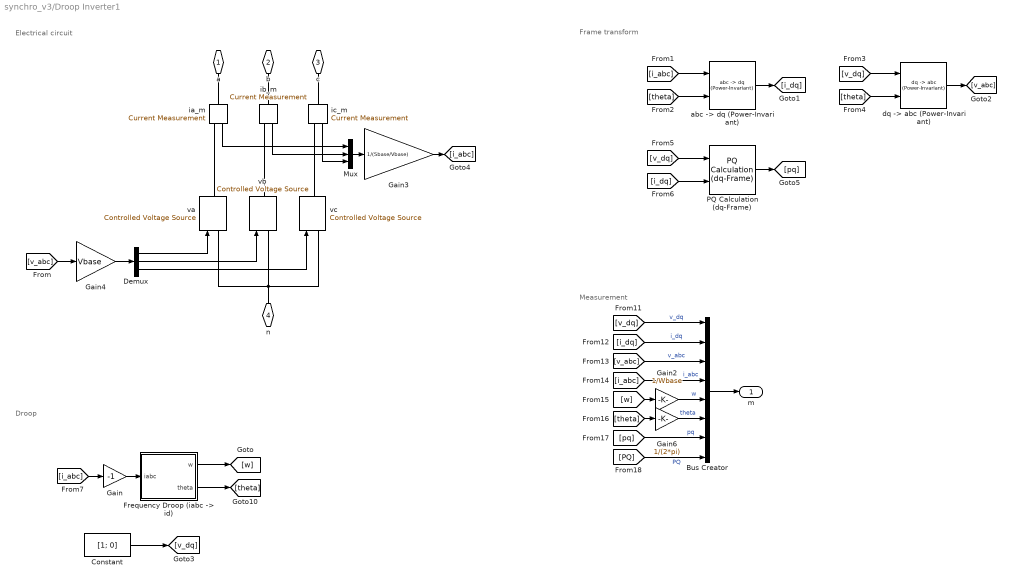
== system synchro_v3/Droop Inverter1 ==
  note: Measurement
  note: Droop
  note: Frame transform
  note: Electrical circuit
  Bus Creator : BusCreator  Inputs=8
  Constant : Constant  Value=[1; 0]
  Demux : Demux  Outputs=3
  "Frequency Droop (iabc -> id)" : Subsystem  AncestorBlock=|  mask{Ts=Ts, Sbase=Sbase, Vbase=Vbase, Wbase=Wbase, m=m, w_tau=w_droop, theta0=0, i0=0, w0=1}
      | SimplexPS/Frequency Droop
      | (iabc -> id)
      mask prompts: Ts "Ts (s), samping period"; Sbase "Sbase (VA), base power"; Vbase "Vbase (V), base voltage"; Wbase "Wbase (rad/s), base angular frequency"; m "m (pu), droop gain"; w_tau "w_tau (rad/s), low-pass filter bandwidth"; theta0 "theta0 (rad), initial angle"; i0 "i0 (pu), current setting point"; w0 "w0 (pu), frequency setting point"
  Gain : Gain  Gain=-1
  Gain2 : Gain  Gain=1/Wbase
  Gain3 : Gain  Gain=1/(Sbase/Vbase)
  Gain4 : Gain  Gain=Vbase
  Gain6 : Gain  Gain=1/(2*pi)
  Mux : Mux  Inputs=3
  PQ Calculation (dq-Frame) : SimplexPS/PQ Calculation (dq-Frame)  SystemSampleTime=-1  VariantActivationTime=update diagram  Latency=0  AutoFrameSizeCalculation=off
      settings: SourceProductName=Simplex Power Systems
  "abc -> dq (Power-Invariant)" : SimplexPS/abc -> dq (Power-Invariant)  SystemSampleTime=-1  VariantActivationTime=update diagram  Latency=0  AutoFrameSizeCalculation=off
      settings: SourceProductName=Simplex Power Systems
  "dq -> abc (Power-Invariant)" : SimplexPS/dq -> abc (Power-Invariant)  SystemSampleTime=-1  VariantActivationTime=update diagram  Latency=0  AutoFrameSizeCalculation=off
      settings: SourceProductName=Simplex Power Systems
  ia_m : powerlib/Measurements/Current Measurement  PhasorSimulation=off  OutputType=Complex  PSBequivalent=0
  ib_m : powerlib/Measurements/Current Measurement  PhasorSimulation=off  OutputType=Complex  PSBequivalent=0
  ic_m : powerlib/Measurements/Current Measurement  PhasorSimulation=off  OutputType=Complex  PSBequivalent=0
  va : powerlib/Electrical Sources/Controlled Voltage Source  Initialize=on  Source_Type=AC  Amplitude=0  Phase=0  Frequency=0  Measurements=None
  vb : powerlib/Electrical Sources/Controlled Voltage Source  Initialize=on  Source_Type=AC  Amplitude=0  Phase=0  Frequency=0  Measurements=None
  vc : powerlib/Electrical Sources/Controlled Voltage Source  Initialize=on  Source_Type=AC  Amplitude=0  Phase=0  Frequency=0  Measurements=None
  a : PMIOPort  Side=Left
  b : PMIOPort  Port=2  Side=Left
  c : PMIOPort  Port=3  Side=Left
  n : PMIOPort  Port=4  Side=Left
  m : Outport
  wires:
  ic_m/1 -> Mux/3
  ia_m/1 -> Mux/1
  ib_m/1 -> Mux/2
  Demux/1 -> va/1
  Demux/2 -> vb/1
  Demux/3 -> vc/1
  [i_abc] -> "abc -> dq (Power-Invariant)"/1
  [theta] -> "abc -> dq (Power-Invariant)"/2
  "abc -> dq (Power-Invariant)"/1 -> [i_dq]
  [v_dq] -> "dq -> abc (Power-Invariant)"/1
  [theta] -> "dq -> abc (Power-Invariant)"/2
  "dq -> abc (Power-Invariant)"/1 -> [v_abc]
  [v_dq] -> Bus Creator/1  "v_dq"
  [v_abc] -> Bus Creator/3  "v_abc"
  [i_abc] -> Bus Creator/4  "i_abc"
  [pq] -> Bus Creator/7  "pq"
  [PQ] -> Bus Creator/8  "PQ"
  Bus Creator/1 -> m/1
  [w] -> Gain2/1
  Gain2/1 -> Bus Creator/5  "w"
  Mux/1 -> Gain3/1
  Gain3/1 -> [i_abc]
  [v_abc] -> Gain4/1
  Gain4/1 -> Demux/1
  [theta] -> Gain6/1
  Gain6/1 -> Bus Creator/6  "theta"
  "Frequency Droop (iabc -> id)"/2(theta) -> [theta]
  [i_abc] -> Gain/1
  "Frequency Droop (iabc -> id)"/1(w) -> [w]
  Constant/1 -> [v_dq]
  [i_dq] -> Bus Creator/2  "i_dq"
  [v_dq] -> PQ Calculation (dq-Frame)/1
  [i_dq] -> PQ Calculation (dq-Frame)/2
  PQ Calculation (dq-Frame)/1 -> [pq]
  Gain/1 -> "Frequency Droop (iabc -> id)"/1(iabc)
  connections:
  ia_m/RConn1 -- va/RConn1
  ia_m/LConn1 -- a/RConn1
  ib_m/RConn1 -- vb/RConn1
  ic_m/RConn1 -- vc/RConn1
  va/LConn1 -- vb/LConn1 -- vc/LConn1 -- n/RConn1
  ib_m/LConn1 -- b/RConn1
  ic_m/LConn1 -- c/RConn1

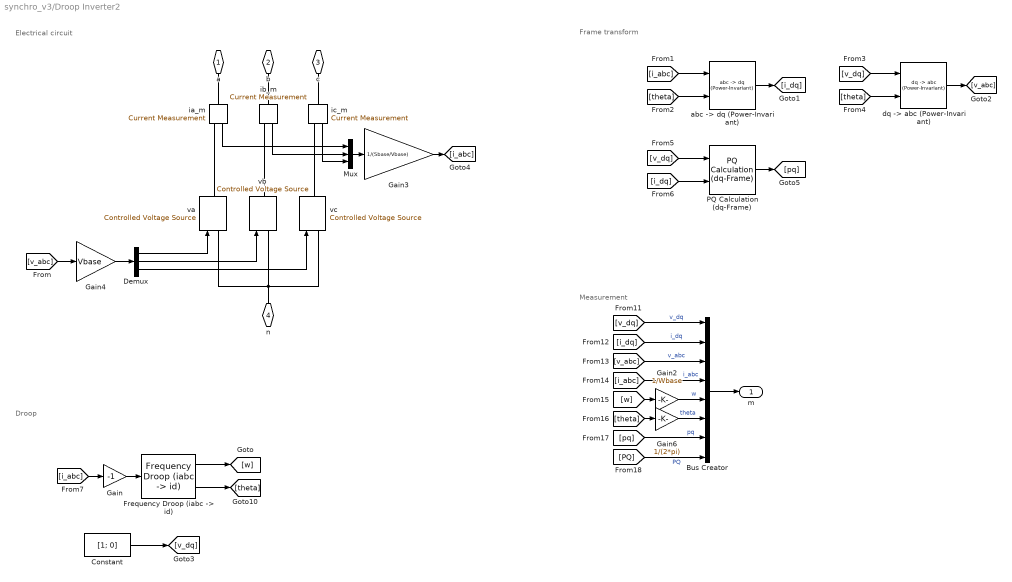
== system synchro_v3/Droop Inverter2 ==
  note: Measurement
  note: Droop
  note: Frame transform
  note: Electrical circuit
  Bus Creator : BusCreator  Inputs=8
  Constant : Constant  Value=[1; 0]
  Demux : Demux  Outputs=3
  "Frequency Droop (iabc -> id)" : SimplexPS/Frequency Droop (iabc -> id)  Ts=Ts  Sbase=Sbase  Vbase=Vbase  Wbase=Wbase  m=m  w_tau=w_droop  theta0=0  i0=0  w0=1
      settings: SourceProductName=Simplex Power Systems
  Gain : Gain  Gain=-1
  Gain2 : Gain  Gain=1/Wbase
  Gain3 : Gain  Gain=1/(Sbase/Vbase)
  Gain4 : Gain  Gain=Vbase
  Gain6 : Gain  Gain=1/(2*pi)
  Mux : Mux  Inputs=3
  PQ Calculation (dq-Frame) : SimplexPS/PQ Calculation (dq-Frame)  SystemSampleTime=-1  VariantActivationTime=update diagram  Latency=0  AutoFrameSizeCalculation=off
      settings: SourceProductName=Simplex Power Systems
  "abc -> dq (Power-Invariant)" : SimplexPS/abc -> dq (Power-Invariant)  SystemSampleTime=-1  VariantActivationTime=update diagram  Latency=0  AutoFrameSizeCalculation=off
      settings: SourceProductName=Simplex Power Systems
  "dq -> abc (Power-Invariant)" : SimplexPS/dq -> abc (Power-Invariant)  SystemSampleTime=-1  VariantActivationTime=update diagram  Latency=0  AutoFrameSizeCalculation=off
      settings: SourceProductName=Simplex Power Systems
  ia_m : powerlib/Measurements/Current Measurement  PhasorSimulation=off  OutputType=Complex  PSBequivalent=0
  ib_m : powerlib/Measurements/Current Measurement  PhasorSimulation=off  OutputType=Complex  PSBequivalent=0
  ic_m : powerlib/Measurements/Current Measurement  PhasorSimulation=off  OutputType=Complex  PSBequivalent=0
  va : powerlib/Electrical Sources/Controlled Voltage Source  Initialize=on  Source_Type=AC  Amplitude=0  Phase=0  Frequency=0  Measurements=None
  vb : powerlib/Electrical Sources/Controlled Voltage Source  Initialize=on  Source_Type=AC  Amplitude=0  Phase=0  Frequency=0  Measurements=None
  vc : powerlib/Electrical Sources/Controlled Voltage Source  Initialize=on  Source_Type=AC  Amplitude=0  Phase=0  Frequency=0  Measurements=None
  a : PMIOPort  Side=Left
  b : PMIOPort  Port=2  Side=Left
  c : PMIOPort  Port=3  Side=Left
  n : PMIOPort  Port=4  Side=Left
  m : Outport
  wires:
  ic_m/1 -> Mux/3
  ia_m/1 -> Mux/1
  ib_m/1 -> Mux/2
  Demux/1 -> va/1
  Demux/2 -> vb/1
  Demux/3 -> vc/1
  [i_abc] -> "abc -> dq (Power-Invariant)"/1
  [theta] -> "abc -> dq (Power-Invariant)"/2
  "abc -> dq (Power-Invariant)"/1 -> [i_dq]
  [v_dq] -> "dq -> abc (Power-Invariant)"/1
  [theta] -> "dq -> abc (Power-Invariant)"/2
  "dq -> abc (Power-Invariant)"/1 -> [v_abc]
  [v_dq] -> Bus Creator/1  "v_dq"
  [v_abc] -> Bus Creator/3  "v_abc"
  [i_abc] -> Bus Creator/4  "i_abc"
  [pq] -> Bus Creator/7  "pq"
  [PQ] -> Bus Creator/8  "PQ"
  Bus Creator/1 -> m/1
  [w] -> Gain2/1
  Gain2/1 -> Bus Creator/5  "w"
  Mux/1 -> Gain3/1
  Gain3/1 -> [i_abc]
  [v_abc] -> Gain4/1
  Gain4/1 -> Demux/1
  [theta] -> Gain6/1
  Gain6/1 -> Bus Creator/6  "theta"
  "Frequency Droop (iabc -> id)"/2 -> [theta]
  [i_abc] -> Gain/1
  "Frequency Droop (iabc -> id)"/1 -> [w]
  Constant/1 -> [v_dq]
  [i_dq] -> Bus Creator/2  "i_dq"
  [v_dq] -> PQ Calculation (dq-Frame)/1
  [i_dq] -> PQ Calculation (dq-Frame)/2
  PQ Calculation (dq-Frame)/1 -> [pq]
  Gain/1 -> "Frequency Droop (iabc -> id)"/1
  connections:
  ia_m/RConn1 -- va/RConn1
  ia_m/LConn1 -- a/RConn1
  ib_m/RConn1 -- vb/RConn1
  ic_m/RConn1 -- vc/RConn1
  va/LConn1 -- vb/LConn1 -- vc/LConn1 -- n/RConn1
  ib_m/LConn1 -- b/RConn1
  ic_m/LConn1 -- c/RConn1

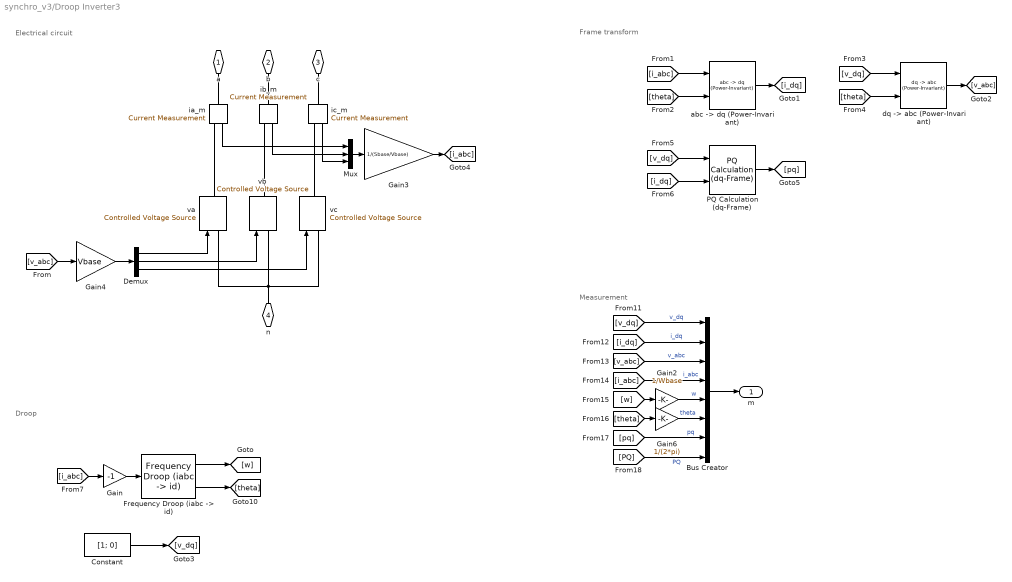
== system synchro_v3/Droop Inverter3 ==
  note: Measurement
  note: Droop
  note: Frame transform
  note: Electrical circuit
  Bus Creator : BusCreator  Inputs=8
  Constant : Constant  Value=[1; 0]
  Demux : Demux  Outputs=3
  "Frequency Droop (iabc -> id)" : SimplexPS/Frequency Droop (iabc -> id)  Ts=Ts  Sbase=Sbase  Vbase=Vbase  Wbase=Wbase  m=m  w_tau=w_droop  theta0=0  i0=0  w0=1
      settings: SourceProductName=Simplex Power Systems
  Gain : Gain  Gain=-1
  Gain2 : Gain  Gain=1/Wbase
  Gain3 : Gain  Gain=1/(Sbase/Vbase)
  Gain4 : Gain  Gain=Vbase
  Gain6 : Gain  Gain=1/(2*pi)
  Mux : Mux  Inputs=3
  PQ Calculation (dq-Frame) : SimplexPS/PQ Calculation (dq-Frame)  SystemSampleTime=-1  VariantActivationTime=update diagram  Latency=0  AutoFrameSizeCalculation=off
      settings: SourceProductName=Simplex Power Systems
  "abc -> dq (Power-Invariant)" : SimplexPS/abc -> dq (Power-Invariant)  SystemSampleTime=-1  VariantActivationTime=update diagram  Latency=0  AutoFrameSizeCalculation=off
      settings: SourceProductName=Simplex Power Systems
  "dq -> abc (Power-Invariant)" : SimplexPS/dq -> abc (Power-Invariant)  SystemSampleTime=-1  VariantActivationTime=update diagram  Latency=0  AutoFrameSizeCalculation=off
      settings: SourceProductName=Simplex Power Systems
  ia_m : powerlib/Measurements/Current Measurement  PhasorSimulation=off  OutputType=Complex  PSBequivalent=0
  ib_m : powerlib/Measurements/Current Measurement  PhasorSimulation=off  OutputType=Complex  PSBequivalent=0
  ic_m : powerlib/Measurements/Current Measurement  PhasorSimulation=off  OutputType=Complex  PSBequivalent=0
  va : powerlib/Electrical Sources/Controlled Voltage Source  Initialize=on  Source_Type=AC  Amplitude=0  Phase=0  Frequency=0  Measurements=None
  vb : powerlib/Electrical Sources/Controlled Voltage Source  Initialize=on  Source_Type=AC  Amplitude=0  Phase=0  Frequency=0  Measurements=None
  vc : powerlib/Electrical Sources/Controlled Voltage Source  Initialize=on  Source_Type=AC  Amplitude=0  Phase=0  Frequency=0  Measurements=None
  a : PMIOPort  Side=Left
  b : PMIOPort  Port=2  Side=Left
  c : PMIOPort  Port=3  Side=Left
  n : PMIOPort  Port=4  Side=Left
  m : Outport
  wires:
  ic_m/1 -> Mux/3
  ia_m/1 -> Mux/1
  ib_m/1 -> Mux/2
  Demux/1 -> va/1
  Demux/2 -> vb/1
  Demux/3 -> vc/1
  [i_abc] -> "abc -> dq (Power-Invariant)"/1
  [theta] -> "abc -> dq (Power-Invariant)"/2
  "abc -> dq (Power-Invariant)"/1 -> [i_dq]
  [v_dq] -> "dq -> abc (Power-Invariant)"/1
  [theta] -> "dq -> abc (Power-Invariant)"/2
  "dq -> abc (Power-Invariant)"/1 -> [v_abc]
  [v_dq] -> Bus Creator/1  "v_dq"
  [v_abc] -> Bus Creator/3  "v_abc"
  [i_abc] -> Bus Creator/4  "i_abc"
  [pq] -> Bus Creator/7  "pq"
  [PQ] -> Bus Creator/8  "PQ"
  Bus Creator/1 -> m/1
  [w] -> Gain2/1
  Gain2/1 -> Bus Creator/5  "w"
  Mux/1 -> Gain3/1
  Gain3/1 -> [i_abc]
  [v_abc] -> Gain4/1
  Gain4/1 -> Demux/1
  [theta] -> Gain6/1
  Gain6/1 -> Bus Creator/6  "theta"
  "Frequency Droop (iabc -> id)"/2 -> [theta]
  [i_abc] -> Gain/1
  "Frequency Droop (iabc -> id)"/1 -> [w]
  Constant/1 -> [v_dq]
  [i_dq] -> Bus Creator/2  "i_dq"
  [v_dq] -> PQ Calculation (dq-Frame)/1
  [i_dq] -> PQ Calculation (dq-Frame)/2
  PQ Calculation (dq-Frame)/1 -> [pq]
  Gain/1 -> "Frequency Droop (iabc -> id)"/1
  connections:
  ia_m/RConn1 -- va/RConn1
  ia_m/LConn1 -- a/RConn1
  ib_m/RConn1 -- vb/RConn1
  ic_m/RConn1 -- vc/RConn1
  va/LConn1 -- vb/LConn1 -- vc/LConn1 -- n/RConn1
  ib_m/LConn1 -- b/RConn1
  ic_m/LConn1 -- c/RConn1

== system synchro_v3/Frequency Droop (id) ==
  iabc : Inport
  Constant : Constant  Value=W0
  Constant2 : Constant  Value=theta0
  Constant4 : Constant  Value=2*pi
  Constant6 : Constant  Value=P0
  Demux1 : Demux  Outputs=2
  Discrete-Time Integrator : DiscreteIntegrator  SampleTime=Ts  ICPrevOutput=DiscIntNeverNeededParam  ICPrevScaledInput=DiscIntNeverNeededParam
  Filter p : DiscreteTransferFcn  Commented=on  Numerator=w_tau*Ts  Denominator=[1 ((w_tau*Ts)-1)]  SampleTime=Ts
  Gain : Gain  Gain=1/(2*pi)
  Gain1 : Gain  Gain=1/(Sbase/Vbase)
  Gain2 : Gain  Gain=m
  Gain3 : Gain  Gain=Wbase
  Gain4 : Gain  Gain=1/Wbase
  Math Function1 : Math  Operator=mod  SignedPower=on  SaturateOnIntegerOverflow=on
  Root Mean Squre : SimplexPS/Root Mean Squre  SystemSampleTime=-1  VariantActivationTime=update diagram  Latency=0  AutoFrameSizeCalculation=off
      settings: SourceProductName=Simplex Power Systems
  Scope : Scope
  Scope2 : Scope  NumInputPorts=4
  Sum : Sum
  Sum1 : Sum
  Sum2 : Sum  Inputs=+-
  "abc -> dq (Power-Invariant)" : SimplexPS/abc -> dq (Power-Invariant)  SystemSampleTime=-1  VariantActivationTime=update diagram  Latency=0  AutoFrameSizeCalculation=off
      settings: SourceProductName=Simplex Power Systems
  w : Outport
  freq : Outport  Port=2
  theta : Outport  Port=3
  wires:
  Sum1/1 -> Math Function1/1
  Constant2/1 -> Sum1/2
  Math Function1/1 -> [theta], "abc -> dq (Power-Invariant)"/2, theta/1
  Gain2/1 -> Sum/1
  Discrete-Time Integrator/1 -> Sum1/1
  Gain1/1 -> Sum2/2
  Constant/1 -> Sum/2
  "abc -> dq (Power-Invariant)"/1 -> Demux1/1
  Constant4/1 -> Math Function1/2
  iabc/1 -> "abc -> dq (Power-Invariant)"/1
  Demux1/1 -> Gain1/1, [id]  "id"
  Constant6/1 -> Sum2/1
  Sum2/1 -> Gain2/1
  Gain/1 -> freq/1
  Sum/1 -> Gain3/1
  Gain3/1 -> [w], w/1, Gain/1, Discrete-Time Integrator/1
  Demux1/2 -> [iq]
  [id] -> Root Mean Squre/1, Scope2/1  "id"
  [iq] -> Root Mean Squre/2, Scope2/2  "iq"
  [w] -> Gain4/1  "w"
  [theta] -> Scope2/4  "theta"
  Gain4/1 -> Scope2/3  "wpu"
  Root Mean Squre/1 -> Scope/1

== system synchro_v3/Frequency Droop (iq) ==
  iabc : Inport
  Constant : Constant  Value=W0
  Constant2 : Constant  Value=theta0
  Constant4 : Constant  Value=2*pi
  Constant6 : Constant  Value=P0
  Demux1 : Demux  Outputs=2
  Discrete-Time Integrator : DiscreteIntegrator  SampleTime=Ts  ICPrevOutput=DiscIntNeverNeededParam  ICPrevScaledInput=DiscIntNeverNeededParam
  Filter p : DiscreteTransferFcn  Numerator=w_tau*Ts  Denominator=[1 ((w_tau*Ts)-1)]  SampleTime=Ts
  Gain : Gain  Gain=1/(2*pi)
  Gain1 : Gain  Gain=1/(Sbase/Vbase)
  Gain2 : Gain  Gain=m
  Gain3 : Gain  Gain=Wbase
  Gain4 : Gain  Gain=-1
  Math Function1 : Math  Operator=mod  SignedPower=on  SaturateOnIntegerOverflow=on
  Scope : Scope
  Sum : Sum
  Sum1 : Sum
  Sum2 : Sum  Inputs=+-
  "abc -> dq (Power-Invariant)" : SimplexPS/abc -> dq (Power-Invariant)  SystemSampleTime=-1  VariantActivationTime=update diagram  Latency=0  AutoFrameSizeCalculation=off
      settings: SourceProductName=Simplex Power Systems
  w : Outport
  freq : Outport  Port=2
  theta : Outport  Port=3
  wires:
  Demux1/2 -> Gain4/1
  Gain3/1 -> Discrete-Time Integrator/1, Gain/1, w/1
  Sum/1 -> Gain3/1
  Gain/1 -> freq/1
  Sum2/1 -> Gain2/1
  Constant6/1 -> Sum2/1
  Gain1/1 -> Scope/1, Filter p/1
  iabc/1 -> "abc -> dq (Power-Invariant)"/1
  Constant4/1 -> Math Function1/2
  "abc -> dq (Power-Invariant)"/1 -> Demux1/1
  Constant/1 -> Sum/2
  Filter p/1 -> Sum2/2
  Discrete-Time Integrator/1 -> Sum1/1
  Gain2/1 -> Sum/1
  Math Function1/1 -> "abc -> dq (Power-Invariant)"/2, theta/1
  Constant2/1 -> Sum1/2
  Sum1/1 -> Math Function1/1
  Gain4/1 -> Gain1/1

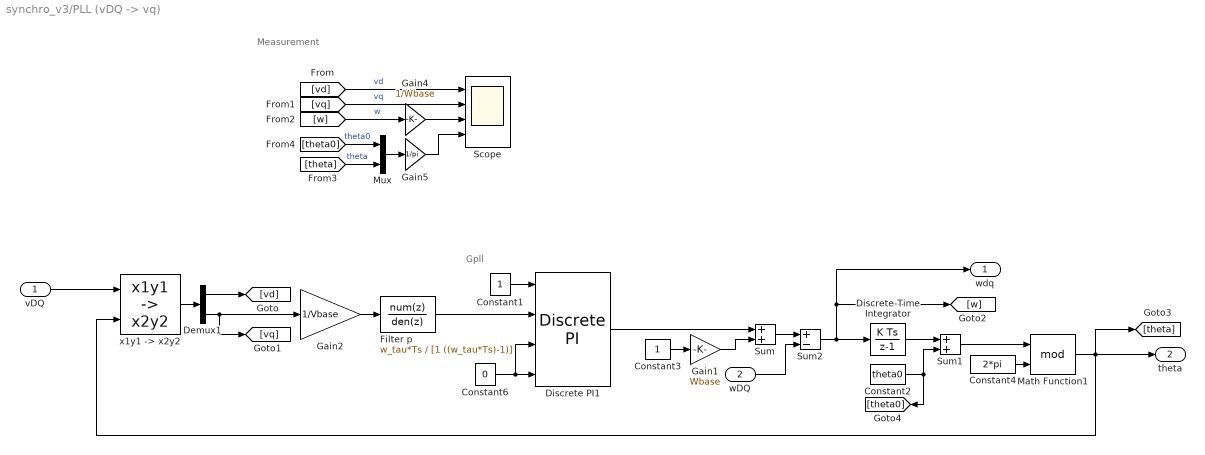
== system synchro_v3/PLL (vDQ -> vq) ==
  note: Gpll
  note: Measurement
  vDQ : Inport
  wDQ : Inport  Port=2
  Constant1 : Constant
  Constant2 : Constant  Value=theta0
  Constant3 : Constant
  Constant4 : Constant  Value=2*pi
  Constant6 : Constant  Value=0
  Demux1 : Demux  Outputs=2
  Discrete PI1 : SimplexPS/Discrete PI  Kp=w_pll  Ki=w_pll*w_pll/4  xmax=inf  xmin=-inf  Ts=Ts
      settings: SourceProductName=Simplex Power Systems
  Discrete-Time Integrator : DiscreteIntegrator  SampleTime=Ts  ICPrevOutput=DiscIntNeverNeededParam  ICPrevScaledInput=DiscIntNeverNeededParam
  Filter p : DiscreteTransferFcn  Numerator=w_tau*Ts  Denominator=[1 ((w_tau*Ts)-1)]  SampleTime=Ts
  Gain1 : Gain  Gain=Wbase
  Gain2 : Gain  Gain=1/Vbase
  Gain4 : Gain  Gain=1/Wbase
  Gain5 : Gain  Gain=1/pi
  Math Function1 : Math  Operator=mod  SignedPower=on  SaturateOnIntegerOverflow=on
  Mux : Mux  Inputs=2
  Scope : Scope  NumInputPorts=4
  Sum : Sum
  Sum1 : Sum
  Sum2 : Sum  Inputs=+-
  "x1y1 -> x2y2" : SimplexPS/x1y1 -> x2y2  SystemSampleTime=-1  VariantActivationTime=update diagram  Latency=0  AutoFrameSizeCalculation=off
      settings: SourceProductName=Simplex Power Systems
  wdq : Outport
  theta : Outport  Port=2
  wires:
  [theta0] -> Mux/1  "theta0"
  Constant2/1 -> [theta0], Sum1/2
  Math Function1/1 -> "x1y1 -> x2y2"/2, theta/1, [theta]
  Sum1/1 -> Math Function1/1
  Demux1/2 -> [vq], Gain2/1
  vDQ/1 -> "x1y1 -> x2y2"/1
  Discrete-Time Integrator/1 -> Sum1/1
  Gain2/1 -> Filter p/1
  [vd] -> Scope/1  "vd"
  Mux/1 -> Gain5/1
  Discrete PI1/1 -> Sum/1
  "x1y1 -> x2y2"/1 -> Demux1/1
  [w] -> Gain4/1  "w"
  Constant4/1 -> Math Function1/2
  [theta] -> Mux/2  "theta"
  Demux1/1 -> [vd]
  Gain5/1 -> Scope/4
  Constant1/1 -> Discrete PI1/1
  Gain4/1 -> Scope/3
  Gain1/1 -> Sum/2
  Constant3/1 -> Gain1/1
  [vq] -> Scope/2  "vq"
  Filter p/1 -> Discrete PI1/2
  Constant6/1 -> Discrete PI1/4, Discrete PI1/3
  Sum/1 -> Sum2/1
  Sum2/1 -> [w], wdq/1, Discrete-Time Integrator/1
  wDQ/1 -> Sum2/2

== system synchro_v3/PLL (vDQ -> vq)1 ==
  note: Gpll
  note: Measurement
  vDQ : Inport
  wDQ : Inport  Port=2
  Constant1 : Constant
  Constant2 : Constant  Value=theta0
  Constant3 : Constant
  Constant4 : Constant  Value=2*pi
  Constant6 : Constant  Value=0
  Demux1 : Demux  Outputs=2
  Discrete PI1 : SimplexPS/Discrete PI  Kp=w_pll  Ki=w_pll*w_pll/4  xmax=inf  xmin=-inf  Ts=Ts
      settings: SourceProductName=Simplex Power Systems
  Discrete-Time Integrator : DiscreteIntegrator  SampleTime=Ts  ICPrevOutput=DiscIntNeverNeededParam  ICPrevScaledInput=DiscIntNeverNeededParam
  Filter p : DiscreteTransferFcn  Numerator=w_tau*Ts  Denominator=[1 ((w_tau*Ts)-1)]  SampleTime=Ts
  Gain1 : Gain  Gain=Wbase
  Gain2 : Gain  Gain=1/Vbase
  Gain4 : Gain  Gain=1/Wbase
  Gain5 : Gain  Gain=1/pi
  Math Function1 : Math  Operator=mod  SignedPower=on  SaturateOnIntegerOverflow=on
  Mux : Mux  Inputs=2
  Scope : Scope  NumInputPorts=4
  Sum : Sum
  Sum1 : Sum
  Sum2 : Sum  Inputs=+-
  "x1y1 -> x2y2" : SimplexPS/x1y1 -> x2y2  SystemSampleTime=-1  VariantActivationTime=update diagram  Latency=0  AutoFrameSizeCalculation=off
      settings: SourceProductName=Simplex Power Systems
  wdq : Outport
  theta : Outport  Port=2
  wires:
  [theta0] -> Mux/1  "theta0"
  Constant2/1 -> [theta0], Sum1/2
  Math Function1/1 -> "x1y1 -> x2y2"/2, theta/1, [theta]
  Sum1/1 -> Math Function1/1
  Demux1/2 -> [vq], Gain2/1
  vDQ/1 -> "x1y1 -> x2y2"/1
  Discrete-Time Integrator/1 -> Sum1/1
  Gain2/1 -> Filter p/1
  [vd] -> Scope/1  "vd"
  Mux/1 -> Gain5/1
  Discrete PI1/1 -> Sum/1
  "x1y1 -> x2y2"/1 -> Demux1/1
  [w] -> Gain4/1  "w"
  Constant4/1 -> Math Function1/2
  [theta] -> Mux/2  "theta"
  Demux1/1 -> [vd]
  Gain5/1 -> Scope/4
  Constant1/1 -> Discrete PI1/1
  Gain4/1 -> Scope/3
  Gain1/1 -> Sum/2
  Constant3/1 -> Gain1/1
  [vq] -> Scope/2  "vq"
  Filter p/1 -> Discrete PI1/2
  Constant6/1 -> Discrete PI1/4, Discrete PI1/3
  Sum/1 -> Sum2/1
  Sum2/1 -> [w], wdq/1, Discrete-Time Integrator/1
  wDQ/1 -> Sum2/2

== system synchro_v3/PLL (vabc -> vq) ==
  note: Measurement
  note: Gpll
  vabc : Inport
  Constant1 : Constant
  Constant2 : Constant  Value=theta0
  Constant3 : Constant
  Constant4 : Constant  Value=2*pi
  Constant6 : Constant  Value=0
  Demux1 : Demux  Outputs=2
  Discrete PI : SimplexPS/Discrete PI  Kp=w_pll  Ki=w_pll*w_pll/4  xmax=inf  xmin=-inf  Ts=Ts
      settings: SourceProductName=Simplex Power Systems
  Discrete-Time Integrator : DiscreteIntegrator  SampleTime=Ts  ICPrevOutput=DiscIntNeverNeededParam  ICPrevScaledInput=DiscIntNeverNeededParam
  Filter p : DiscreteTransferFcn  Numerator=w_tau*Ts  Denominator=[1 ((w_tau*Ts)-1)]  SampleTime=Ts
  Gain1 : Gain  Gain=Wbase
  Gain2 : Gain  Gain=1/Vbase
  Gain4 : Gain  Gain=1/Wbase
  Gain5 : Gain  Gain=1/pi
  Math Function1 : Math  Operator=mod  SignedPower=on  SaturateOnIntegerOverflow=on
  Mux : Mux  Inputs=2
  Scope : Scope  NumInputPorts=4
  Sum : Sum
  Sum1 : Sum
  "abc -> dq (Power-Invariant)" : SimplexPS/abc -> dq (Power-Invariant)  SystemSampleTime=-1  VariantActivationTime=update diagram  Latency=0  AutoFrameSizeCalculation=off
      settings: SourceProductName=Simplex Power Systems
  w : Outport
  theta : Outport  Port=2
  wires:
  vabc/1 -> "abc -> dq (Power-Invariant)"/1
  "abc -> dq (Power-Invariant)"/1 -> Demux1/1
  Constant4/1 -> Math Function1/2
  Gain2/1 -> Filter p/1
  Demux1/2 -> [vq], Gain2/1
  Constant6/1 -> Discrete PI/4, Discrete PI/3
  Constant1/1 -> Discrete PI/1
  Discrete PI/1 -> Sum/1
  Sum/1 -> [w], w/1, Discrete-Time Integrator/1
  Gain1/1 -> Sum/2
  Discrete-Time Integrator/1 -> Sum1/1
  Sum1/1 -> Math Function1/1
  Constant2/1 -> [theta0], Sum1/2
  Filter p/1 -> Discrete PI/2
  [vq] -> Scope/2  "vq"
  Mux/1 -> Gain5/1
  Gain4/1 -> Scope/3
  [w] -> Gain4/1  "w"
  [theta0] -> Mux/1  "theta0"
  [vd] -> Scope/1  "vd"
  Gain5/1 -> Scope/4
  [theta] -> Mux/2  "theta"
  Demux1/1 -> [vd]
  Constant3/1 -> Gain1/1
  Math Function1/1 -> "abc -> dq (Power-Invariant)"/2, [theta], theta/1

== system synchro_v3/PLL (vabc -> vq)1 ==
  note: Measurement
  note: Gpll
  vabc : Inport
  Constant1 : Constant
  Constant2 : Constant  Value=theta0
  Constant3 : Constant
  Constant4 : Constant  Value=2*pi
  Constant6 : Constant  Value=0
  Demux1 : Demux  Outputs=2
  Discrete PI : SimplexPS/Discrete PI  Kp=w_pll  Ki=w_pll*w_pll/4  xmax=inf  xmin=-inf  Ts=Ts
      settings: SourceProductName=Simplex Power Systems
  Discrete-Time Integrator : DiscreteIntegrator  SampleTime=Ts  ICPrevOutput=DiscIntNeverNeededParam  ICPrevScaledInput=DiscIntNeverNeededParam
  Filter p : DiscreteTransferFcn  Numerator=w_tau*Ts  Denominator=[1 ((w_tau*Ts)-1)]  SampleTime=Ts
  Gain1 : Gain  Gain=Wbase
  Gain2 : Gain  Gain=1/Vbase
  Gain4 : Gain  Gain=1/Wbase
  Gain5 : Gain  Gain=1/pi
  Math Function1 : Math  Operator=mod  SignedPower=on  SaturateOnIntegerOverflow=on
  Mux : Mux  Inputs=2
  Scope : Scope  NumInputPorts=4
  Sum : Sum
  Sum1 : Sum
  "abc -> dq (Power-Invariant)" : SimplexPS/abc -> dq (Power-Invariant)  SystemSampleTime=-1  VariantActivationTime=update diagram  Latency=0  AutoFrameSizeCalculation=off
      settings: SourceProductName=Simplex Power Systems
  w : Outport
  theta : Outport  Port=2
  wires:
  vabc/1 -> "abc -> dq (Power-Invariant)"/1
  "abc -> dq (Power-Invariant)"/1 -> Demux1/1
  Constant4/1 -> Math Function1/2
  Gain2/1 -> Filter p/1
  Demux1/2 -> [vq], Gain2/1
  Constant6/1 -> Discrete PI/4, Discrete PI/3
  Constant1/1 -> Discrete PI/1
  Discrete PI/1 -> Sum/1
  Sum/1 -> [w], w/1, Discrete-Time Integrator/1
  Gain1/1 -> Sum/2
  Discrete-Time Integrator/1 -> Sum1/1
  Sum1/1 -> Math Function1/1
  Constant2/1 -> [theta0], Sum1/2
  Filter p/1 -> Discrete PI/2
  [vq] -> Scope/2  "vq"
  Mux/1 -> Gain5/1
  Gain4/1 -> Scope/3
  [w] -> Gain4/1  "w"
  [theta0] -> Mux/1  "theta0"
  [vd] -> Scope/1  "vd"
  Gain5/1 -> Scope/4
  [theta] -> Mux/2  "theta"
  Demux1/1 -> [vd]
  Constant3/1 -> Gain1/1
  Math Function1/1 -> "abc -> dq (Power-Invariant)"/2, [theta], theta/1
